simulink model "lab_2"  (R2023a)
settings: Solver=VariableStepAuto  StartTime=0.0  StopTime=30  RelTol=1e-3
settings Model: Creator=User  LastModifiedBy=User

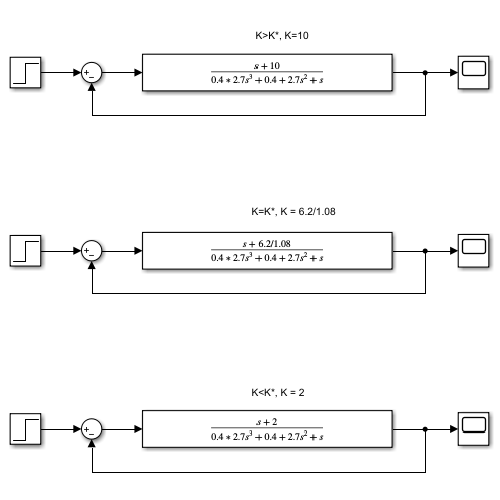
[thumbnail: Simulink's stored preview of the top-level diagram]
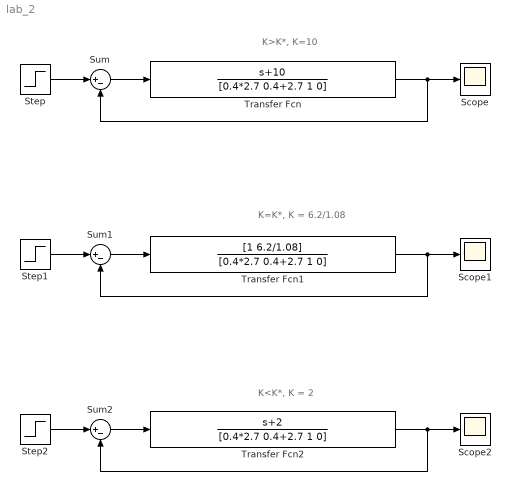
== system lab_2 ==
  note: K>K*, K=10
  note: K=K*, K = 6.2/1.08
  note: K<K*, K = 2
  Scope : Scope
  Scope1 : Scope
  Scope2 : Scope
  Step : Step  SampleTime=0
  Step1 : Step  SampleTime=0
  Step2 : Step  SampleTime=0
  Sum : Sum  Inputs=|+-
  Sum1 : Sum  Inputs=|+-
  Sum2 : Sum  Inputs=|+-
  Transfer Fcn : TransferFcn  Numerator=[1 10]  Denominator=[0.4*2.7 0.4+2.7 1 0]
  Transfer Fcn1 : TransferFcn  Numerator=[1 6.2/1.08]  Denominator=[0.4*2.7 0.4+2.7 1 0]
  Transfer Fcn2 : TransferFcn  Numerator=[1 2]  Denominator=[0.4*2.7 0.4+2.7 1 0]
  wires:
  Step/1 -> Sum/1
  Sum/1 -> Transfer Fcn/1
  Transfer Fcn/1 -> Sum/2, Scope/1
  Step1/1 -> Sum1/1
  Sum1/1 -> Transfer Fcn1/1
  Transfer Fcn1/1 -> Sum1/2, Scope1/1
  Step2/1 -> Sum2/1
  Sum2/1 -> Transfer Fcn2/1
  Transfer Fcn2/1 -> Sum2/2, Scope2/1
